simulink model "mmr_ground_yM"  (R2019a)
settings: Solver=ode4  StartTime=0.0  StopTime=tc  RelTol=1e-1
values from neighbouring files (symbols this model uses):
  g = -9.81    [MMR.m]    (also in MMR_alfa0.m; MMR_alone.m; MMR_hop_zero.m = 9.81)
  k = 2000.0    (= 2000)    [MMR.m]    (also in MMR_alfa0.m = 22500; MMR_alone.m; MMR_hop_zero.m = 8515.125)
  L0 = sqrt(x0*x0 + y0*y0)    [MMR.m]    (also in MMR_alfa0.m; MMR_alone.m)
  Lcol = 0.70    (= 0.7)    [MMR.m]    (also in MMR_alone.m)
  Lhk = 0.28    [MMR.m]    (also in MMR_alfa0.m; MMR_alone.m; MMR_hop_zero.m)
  Lkf = 0.28    [MMR.m]    (also in MMR_alfa0.m; MMR_alone.m; MMR_hop_zero.m)
  m = 3    [MMR.m]    (also in MMR_alfa0.m; MMR_alone.m; MMR_hop_zero.m)
  M = 15    [MMR.m]    (also in MMR_alfa0.m; MMR_alone.m; MMR_hop_zero.m)
  vx0 = vxair( length(vxair) )    [MMR.m]    (also in MMR_alfa0.m = 0; MMR_alone.m)
  vxM0 = vxair( length(vxMair) )    [MMR.m]    (also in MMR_alfa0.m = 0; MMR_alone.m)
  vy0 = vyair( length(vyair) )    [MMR.m]    (also in MMR_alfa0.m = -0.7; MMR_alone.m; MMR_hop_zero.m = -0.613125)
  vyM0 = vyair( length(vyMair) )    [MMR.m]    (also in MMR_alfa0.m = -0.7; MMR_alone.m)
  x0 = Lkf * sin(alfa0 - beta0)    [MMR.m]    (also in MMR_alfa0.m = 0; MMR_alone.m)
  xM0 = x0 + Lhk*sin(alfa0)    [MMR.m]    (also in MMR_alfa0.m = 0; MMR_alone.m = x0 + Lhk*cos(alfa0))
  y0 = Lkf * cos(alfa0 - beta0)    [MMR.m]    (also in MMR_alfa0.m = 0.28; MMR_alone.m; MMR_hop_zero.m = 0.56)
undefined symbols (not defined in the file or in its folder): magnitude
settings Model: Creator=Jesus  LastModifiedBy=Jesus
settings SolverCC: MaxConsecutiveMinStep=3

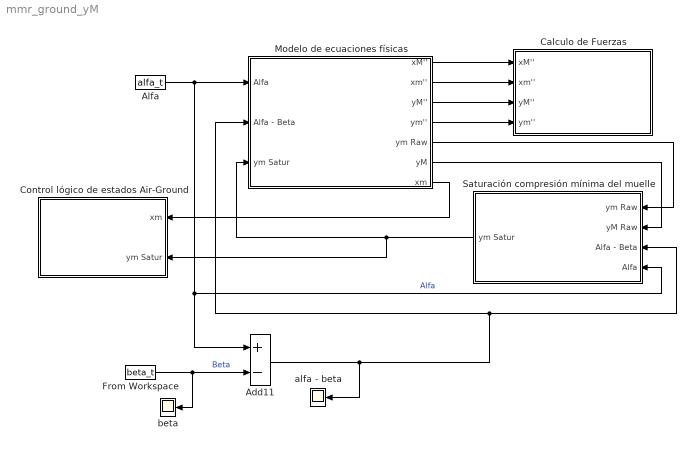
== system mmr_ground_yM ==
  Add11 : Sum  Inputs=+-
  "Alfa " : FromWorkspace  VariableName=alfa_t  SampleTime=0
  Calculo de Fuerzas : Subsystem
  Control lógico de estados Air-Ground : Subsystem
  From Workspace : FromWorkspace  VariableName=beta_t  SampleTime=0
  Modelo de ecuaciones físicas : Subsystem
  Saturación compresión mínima del muelle : Subsystem
  alfa - beta : Scope
  beta : Scope
  wires:
  From Workspace/1 -> beta/1, Add11/2  "Beta"
  "Alfa "/1 -> Add11/1, Saturación compresión mínima del muelle/4(Alfa), Modelo de ecuaciones físicas/1(Alfa)  "Alfa"
  Add11/1 -> alfa - beta/1, Saturación compresión mínima del muelle/3(Alfa - Beta), Modelo de ecuaciones físicas/2(Alfa - Beta)
  Modelo de ecuaciones físicas/1(xM'') -> Calculo de Fuerzas/1(xM'')
  Modelo de ecuaciones físicas/2(xm'') -> Calculo de Fuerzas/2(xm'')
  Modelo de ecuaciones físicas/3(yM'') -> Calculo de Fuerzas/3(yM'')
  Modelo de ecuaciones físicas/4(ym'') -> Calculo de Fuerzas/4(ym'')
  Modelo de ecuaciones físicas/5(ym Raw) -> Saturación compresión mínima del muelle/1(ym Raw)
  Modelo de ecuaciones físicas/6(yM) -> Saturación compresión mínima del muelle/2(yM Raw)
  Saturación compresión mínima del muelle/1(ym Satur) -> Control lógico de estados Air-Ground/2(ym Satur), Modelo de ecuaciones físicas/3(ym Satur)
  Modelo de ecuaciones físicas/7("xm ") -> Control lógico de estados Air-Ground/1(xm)

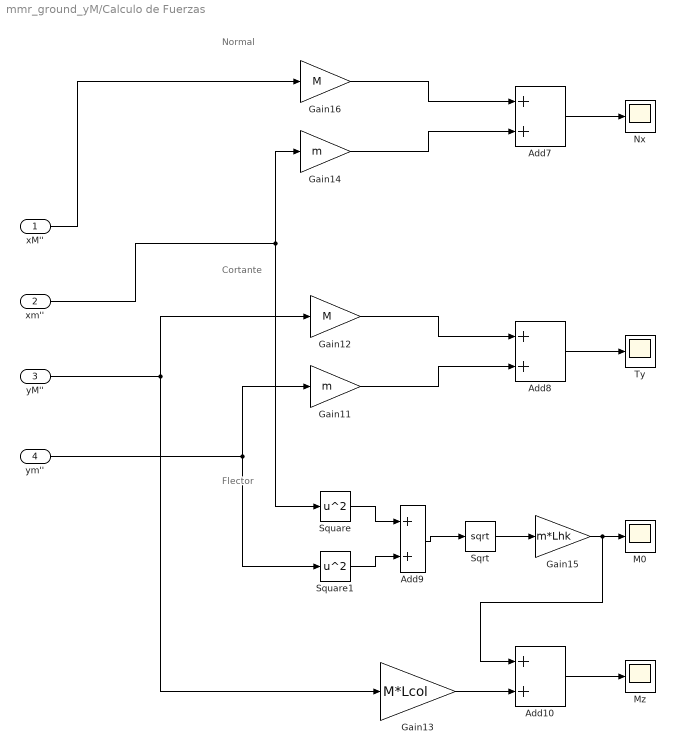
== system mmr_ground_yM/Calculo de Fuerzas ==
  note: Flector
  note: Normal
  note: Cortante
  xM'' : Inport
  xm'' : Inport  Port=2
  yM'' : Inport  Port=3
  ym'' : Inport  Port=4
  Add{7..10} (4 alike) : Sum
  Gain11 : Gain  Gain=m
  Gain12 : Gain  Gain=M
  Gain13 : Gain  Gain=M*Lcol
  Gain14 : Gain  Gain=m
  Gain15 : Gain  Gain=m*Lhk
  Gain16 : Gain  Gain=M
  M0 : Scope
  Mz : Scope
  Nx : Scope
  Sqrt : Sqrt  SaturateOnIntegerOverflow=on
  Square : Math  Operator=square  SaturateOnIntegerOverflow=on
  Square1 : Math  Operator=square  SaturateOnIntegerOverflow=on
  Ty : Scope
  wires:
  Gain11/1 -> Add8/2
  Gain13/1 -> Add10/2
  xM''/1 -> Gain16/1
  Square/1 -> Add9/1
  xm''/1 -> Gain14/1, Square/1
  Sqrt/1 -> Gain15/1
  Add9/1 -> Sqrt/1
  Gain12/1 -> Add8/1
  ym''/1 -> Gain11/1, Square1/1
  Add7/1 -> Nx/1
  Add10/1 -> Mz/1
  Gain15/1 -> Add10/1, M0/1
  Gain16/1 -> Add7/1
  Square1/1 -> Add9/2
  Add8/1 -> Ty/1
  Gain14/1 -> Add7/2
  yM''/1 -> Gain12/1, Gain13/1

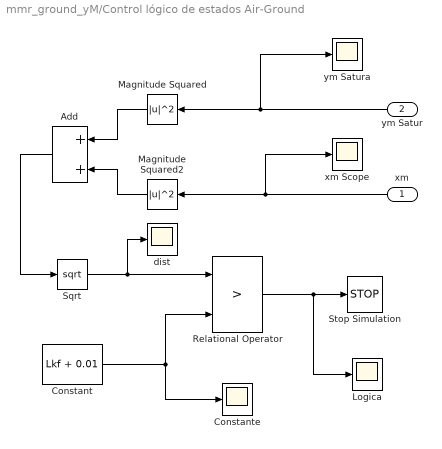
== system mmr_ground_yM/Control lógico de estados Air-Ground ==
  xm : Inport
  ym Satur : Inport  Port=2
  Add : Sum
  Constant : Constant  Value=Lkf + 0.01
  Constante : Scope
  Logica : Scope
  Magnitude Squared : Math  Operator=magnitude^2  SaturateOnIntegerOverflow=on
  Magnitude Squared2 : Math  Operator=magnitude^2  SaturateOnIntegerOverflow=on
  Relational Operator : RelationalOperator  Operator=>  OutDataTypeStr=boolean  RndMeth=Simplest
  Sqrt : Sqrt  SaturateOnIntegerOverflow=on
  Stop Simulation : Stop
  dist : Scope
  xm Scope : Scope
  ym Satura : Scope
  wires:
  Relational Operator/1 -> Logica/1, Stop Simulation/1
  ym Satur/1 -> Magnitude Squared/1, ym Satura/1
  Constant/1 -> Constante/1, Relational Operator/2
  xm/1 -> xm Scope/1, Magnitude Squared2/1
  Sqrt/1 -> dist/1, Relational Operator/1
  Magnitude Squared/1 -> Add/1
  Magnitude Squared2/1 -> Add/2
  Add/1 -> Sqrt/1

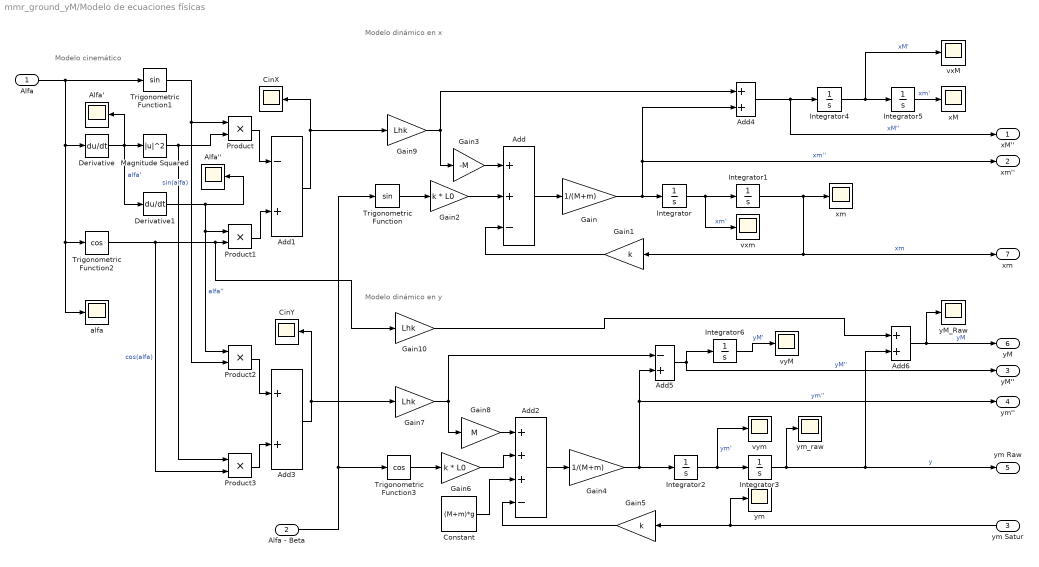
== system mmr_ground_yM/Modelo de ecuaciones físicas ==
  note: Modelo dinámico en x
  note: Modelo dinámico en y
  note: Modelo cinemático
  Alfa : Inport
  Alfa - Beta : Inport  Port=2
  ym Satur : Inport  Port=3
  Add : Sum  Inputs=++-
  Add1 : Sum  Inputs=-+
  Add2 : Sum  Inputs=+++-
  Add3 : Sum
  Add4 : Sum
  Add5 : Sum  Inputs=-+
  Add6 : Sum
  Alfa' : Scope
  Alfa'' : Scope
  CinX : Scope
  CinY : Scope
  Constant : Constant  Value=(M+m)*g
  Derivative : Derivative  CoefficientInTFapproximation=1000
  Derivative1 : Derivative  CoefficientInTFapproximation=1000
  Gain : Gain  Gain=1/(M+m)
  Gain1 : Gain  Gain=k
  Gain10 : Gain  Gain=Lhk
  Gain2 : Gain  Gain=k * L0
  Gain3 : Gain  Gain=-M
  Gain4 : Gain  Gain=1/(M+m)
  Gain5 : Gain  Gain=k
  Gain6 : Gain  Gain=k * L0
  Gain7 : Gain  Gain=Lhk
  Gain8 : Gain  Gain=M
  Gain9 : Gain  Gain=Lhk
  Integrator : Integrator  InitialCondition=vx0
  Integrator1 : Integrator  InitialCondition=x0
  Integrator2 : Integrator  InitialCondition=vy0
  Integrator3 : Integrator  InitialCondition=y0
  Integrator4 : Integrator  InitialCondition=vxM0
  Integrator5 : Integrator  InitialCondition=xM0
  Integrator6 : Integrator  InitialCondition=vyM0
  Magnitude Squared : Math  Operator=magnitude^2  SaturateOnIntegerOverflow=on
  Product{,1..3} (4 alike) : Product
  Trigonometric Function : Trigonometry
  Trigonometric Function1 : Trigonometry
  Trigonometric Function2 : Trigonometry  Operator=cos
  Trigonometric Function3 : Trigonometry  Operator=cos
  alfa : Scope
  "vxM " : Scope
  vxm : Scope
  vyM : Scope
  vym : Scope
  xM : Scope
  xm : Scope
  yM_Raw : Scope
  ym : Scope
  "ym_raw " : Scope
  xM'' : Outport
  xm'' : Outport  Port=2
  yM'' : Outport  Port=3
  ym'' : Outport  Port=4
  ym Raw : Outport  Port=5
  yM : Outport  Port=6
  "xm " : Outport  Port=7
  wires:
  Derivative/1 -> Alfa'/1, Derivative1/1, Magnitude Squared/1  "alfa'"
  Add1/1 -> Gain9/1, CinX/1
  Add4/1 -> Integrator4/1, xM''/1  "xM''"
  Gain4/1 -> Integrator2/1, Add5/2, ym''/1  "ym''"
  Integrator6/1 -> vyM/1  "yM'"
  Gain/1 -> Add4/2, xm''/1, Integrator/1  "xm''"
  Trigonometric Function3/1 -> Gain6/1
  Add2/1 -> Gain4/1
  Integrator3/1 -> "ym_raw "/1, Add6/2, ym Raw/1  "y"
  Gain5/1 -> Add2/4
  Integrator1/1 -> "xm "/1, Gain1/1, xm/1  "xm"
  Trigonometric Function2/1 -> Product3/2, Gain10/1, Product1/2  "cos(alfa)"
  Add3/1 -> Gain7/1, CinY/1
  ym Satur/1 -> ym/1, Gain5/1
  Gain9/1 -> Add4/1, Gain3/1
  Magnitude Squared/1 -> Product3/1, Product/2
  Add/1 -> Gain/1
  Constant/1 -> Add2/3
  Product/1 -> Add1/1
  Product1/1 -> Add1/2
  Alfa - Beta/1 -> Trigonometric Function3/1, Trigonometric Function/1
  Gain7/1 -> Add5/1, Gain8/1
  Alfa/1 -> alfa/1, Trigonometric Function2/1, Derivative/1, Trigonometric Function1/1
  Integrator/1 -> vxm/1, Integrator1/1  "xm'"
  Gain1/1 -> Add/3
  Integrator5/1 -> xM/1  "xm'"
  Add5/1 -> Integrator6/1, yM''/1  "yM''"
  Trigonometric Function1/1 -> Product2/2, Product/1  "sin(alfa)"
  Add6/1 -> yM_Raw/1, yM/1  "yM"
  Derivative1/1 -> Alfa''/1, Product1/1, Product2/1  "alfa''"
  Gain3/1 -> Add/1
  Integrator2/1 -> vym/1, Integrator3/1  "ym'"
  Product2/1 -> Add3/1
  Product3/1 -> Add3/2
  Gain6/1 -> Add2/2
  Gain2/1 -> Add/2
  Trigonometric Function/1 -> Gain2/1
  Integrator4/1 -> Integrator5/1, "vxM "/1  "xM'"
  Gain8/1 -> Add2/1
  Gain10/1 -> Add6/1

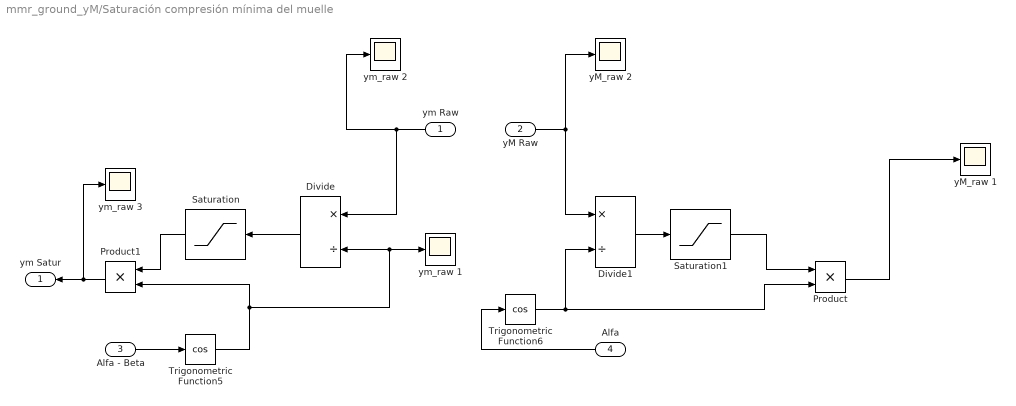
== system mmr_ground_yM/Saturación compresión mínima del muelle ==
  ym Raw : Inport
  yM Raw : Inport  Port=2
  Alfa - Beta : Inport  Port=3
  Alfa : Inport  Port=4
  Divide : Product  Inputs=*/
  Divide1 : Product  Inputs=*/
  Product : Product
  Product1 : Product
  Saturation : Saturate  UpperLimit=inf  LowerLimit=-inf
  Saturation1 : Saturate  UpperLimit=inf  LowerLimit=-inf
  Trigonometric Function5 : Trigonometry  Operator=cos
  Trigonometric Function6 : Trigonometry  Operator=cos
  yM_raw 1 : Scope
  yM_raw 2 : Scope
  ym_raw 1 : Scope
  ym_raw 2 : Scope
  ym_raw 3 : Scope
  ym Satur : Outport
  wires:
  Trigonometric Function5/1 -> Product1/2, Divide/2, ym_raw 1/1
  Divide/1 -> Saturation/1
  Trigonometric Function6/1 -> Divide1/2, Product/2
  yM Raw/1 -> Divide1/1, yM_raw 2/1
  Divide1/1 -> Saturation1/1
  Alfa - Beta/1 -> Trigonometric Function5/1
  ym Raw/1 -> ym_raw 2/1, Divide/1
  Alfa/1 -> Trigonometric Function6/1
  Product/1 -> yM_raw 1/1
  Saturation1/1 -> Product/1
  Saturation/1 -> Product1/1
  Product1/1 -> ym_raw 3/1, ym Satur/1
